simulink model "builder_test"  (R2024a)
settings: Solver=FixedStepDiscrete  StartTime=0.0  StopTime=1  FixedStep=1e-6  RelTol=1e-3  EnableMultiTasking=on
settings Model: Creator=Administrator  LastModifiedBy=Administrator

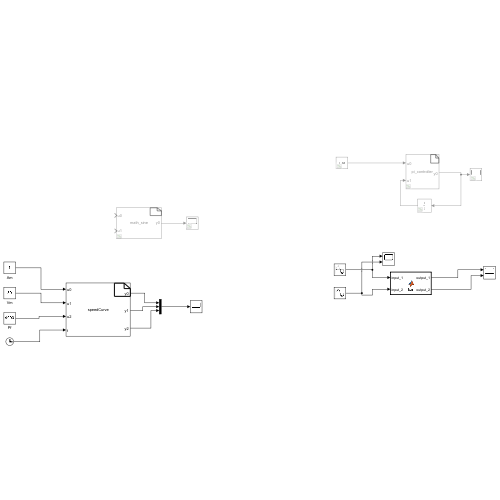
[thumbnail: Simulink's stored preview of the top-level diagram]
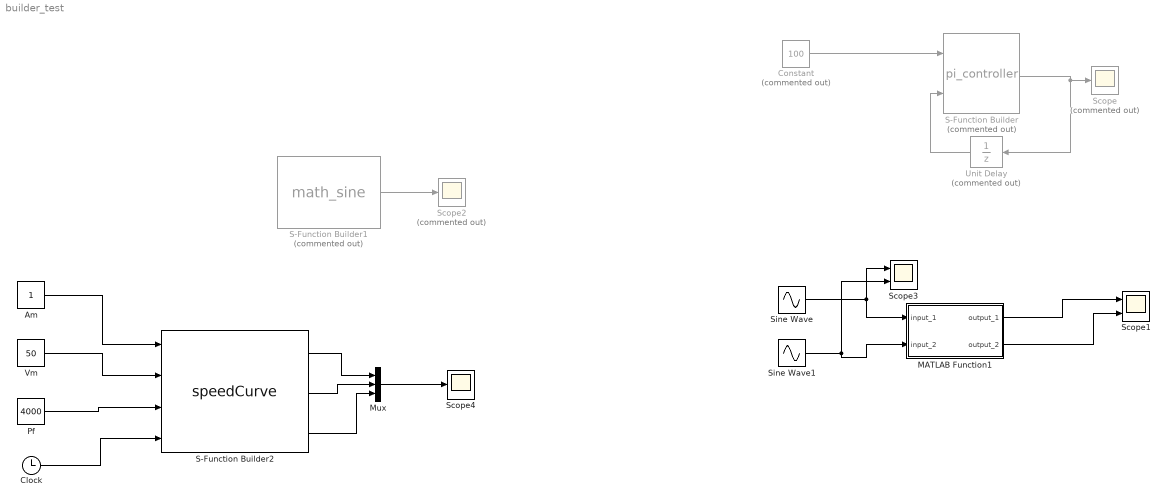
== system builder_test ==
  Am : Constant
  Clock : Clock
  Constant : Constant  Commented=on  Value=100
  MATLAB Function1 : MATLAB Function  TreatAsAtomicUnit=on
  Mux : Mux  Inputs=3
  Pf : Constant  Value=4000
  S-Function Builder : S-Function  Commented=on  FunctionName=pi_controller  SFunctionModules=pi_controller_wrapper.c  SFunctionDeploymentMode=off  EnableBusSupport=off  mask(S-Function Builder){}
      mask help: Simulink:masks:SFunctionBuilder_MD
      mask init:
      | val = [[.9  0.75 0.75 1 1 .9 .9 1]',[1 1 0.75 0.75 .9 .9 1 .9]'];try , sys = get_param(gcb,'SfunBuilderFcnName');if isempty(sys), sys = get_param(gcb,'FunctionName'); end,catch, sys = get_param(gcb,'FunctionName'); end
      settings: CopyFcn=set_param(gcbh,'LinkStatus','none')  OpenFcn=sfunctionwizard(gcbh)
      mask Display:
      | plot(val(:,1),val(:,2))
      | disp(sys)
      | port_label('input',1,sprintf('%s', 'u0'),'interpreter','tex')
      | port_label('input',2,sprintf('%s', 'u1'),'interpreter','tex')
      | port_label('output',1,sprintf('%s', 'y0'),'interpreter','tex')
  S-Function Builder1 : S-Function  Commented=on  FunctionName=math_sine  SFunctionModules=math_sine_wrapper.c  SFunctionDeploymentMode=off  EnableBusSupport=off  mask(S-Function Builder){}
      mask help: Simulink:masks:SFunctionBuilder_MD
      mask init: same as builder_test/S-Function Builder
      settings: CopyFcn=set_param(gcbh,'LinkStatus','none')  OpenFcn=sfunctionwizard(gcbh)
      mask Display: plot(val(:,1),val(:,2)),disp(sys),port_label('input',1,'u0'),port_label('input',2,'u1'),port_label('output',1,'y0')
  S-Function Builder2 : S-Function  FunctionName=speedCurve  SFunctionModules=speedCurve_wrapper.c  SFunctionDeploymentMode=off  EnableBusSupport=off  mask(S-Function Builder){}
      mask help: Simulink:masks:SFunctionBuilder_MD
      mask init: same as builder_test/S-Function Builder
      settings: CopyFcn=set_param(gcbh,'LinkStatus','none')  OpenFcn=sfunctionwizard(gcbh)
      mask Display:
      | plot(val(:,1),val(:,2))
      | disp(sys)
      | port_label('input',1,sprintf('%s', 'u0'),'interpreter','tex')
      | port_label('input',2,sprintf('%s', 'u1'),'interpreter','tex')
      | port_label('input',3,sprintf('%s', 'u2'),'interpreter','tex')
      | port_label('input',4,sprintf('%s', 't'),'interpreter','tex')
      | port_label('output',1,sprintf('%s', 'y0'),'interpreter','tex')
      | port_label('output',2,sprintf('%s', 'y1'),'interpreter','tex')
      | port_label('output',3,sprintf('%s', 'y2'),'interpreter','tex')
  Scope : Scope  Commented=on
  Scope1 : Scope  NumInputPorts=2
  Scope2 : Scope  Commented=on
  Scope3 : Scope  NumInputPorts=2
  Scope4 : Scope
  Sine Wave : Sin  Frequency=2*pi*50  SampleTime=1e-6
  Sine Wave1 : Sin  Frequency=2*pi*50  Phase=pi/2  SampleTime=1e-6
  Unit Delay : UnitDelay  Commented=on  SampleTime=-1  HasFrameUpgradeWarning=on
  Vm : Constant  Value=50
  wires:
  S-Function Builder/1 -> Unit Delay/1, Scope/1
  Constant/1 -> S-Function Builder/1
  Unit Delay/1 -> S-Function Builder/2
  MATLAB Function1/1(output_1) -> Scope1/1
  Sine Wave/1 -> MATLAB Function1/1(input_1), Scope3/1
  Sine Wave1/1 -> MATLAB Function1/2(input_2), Scope3/2
  MATLAB Function1/2(output_2) -> Scope1/2
  S-Function Builder1/1 -> Scope2/1
  Am/1 -> S-Function Builder2/1
  Vm/1 -> S-Function Builder2/2
  Pf/1 -> S-Function Builder2/3
  Clock/1 -> S-Function Builder2/4
  S-Function Builder2/1 -> Mux/1
  S-Function Builder2/2 -> Mux/2
  S-Function Builder2/3 -> Mux/3
  Mux/1 -> Scope4/1

== matlab function builder_test/MATLAB Function1 ==
  data: input_1 input; output_1 output; input_2 input; output_2 output
function [output_1,output_2] = fcn(input_1, input_2)

output_1 = input_1+input_2;
output_2 = input_1-input_2;
